simulink model "v06_arbitrary_coder"  (R2019b)
settings: Solver=FixedStepAuto  StartTime=0.0  StopTime=inf  FixedStep=1  MaxStep=1  RelTol=1e-3
libraries: simulink x3
settings Model: Creator=MARAT  LastModifiedBy=Marat
settings SFSimCC: CustomCodeUndefinedFunction=UseInterfaceOnly
settings ConfigComp: DVTestSuiteOptimization=Auto  DVDetectOutOfBounds=on

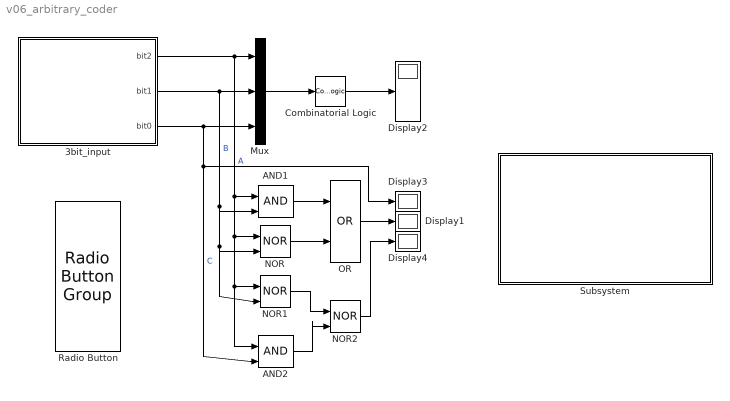
== system v06_arbitrary_coder ==
  3bit_input : Subsystem
      mask Display: image('images\3bit.jpg'); % Use "Edit Image" on toolstrip to change.
  AND1 : Logic  IconShape=distinctive  AllPortsSameDT=off  OutDataTypeStr=boolean
  AND2 : Logic  IconShape=distinctive  AllPortsSameDT=off  OutDataTypeStr=boolean
  Combinatorial Logic : CombinatorialLogic  TruthTable=[0 1 0 ; 1 1 0 ; 0 0 1 ; 1 0 1 ; 0 0 1 ; 1 0 0 ; 0 1 1 ; 1 1 0]
  Display{1..4} (4 alike) : Display
  Mux : Mux  Inputs=3
  NOR : Logic  Operator=NOR  IconShape=distinctive  AllPortsSameDT=off  OutDataTypeStr=boolean
  NOR1 : Logic  Operator=NOR  IconShape=distinctive  AllPortsSameDT=off  OutDataTypeStr=boolean
  NOR2 : Logic  Operator=NOR  IconShape=distinctive  AllPortsSameDT=off  OutDataTypeStr=boolean
  OR : Logic  Operator=OR  IconShape=distinctive  AllPortsSameDT=off  OutDataTypeStr=boolean
  Radio Button : RadioButtonGroup  SelectedLabel=0
      settings: Values={{'0', '1', '2', '3', '4', '5', '6', '7'}, [0 1 2 3 4 5 6 7]}
  Subsystem : Subsystem
      mask Display: image('D:\Work\DS_in_SL\pics\v06\table.png'); % Use "Edit Image" on toolstrip to change.
  wires:
  Mux/1 -> Combinatorial Logic/1
  Combinatorial Logic/1 -> Display2/1
  3bit_input/1(bit2) -> AND2/1, NOR1/1, NOR/1, AND1/1, Mux/1  "A"
  3bit_input/2(bit1) -> NOR1/2, NOR/2, AND1/2, Mux/2  "B"
  3bit_input/3(bit0) -> AND2/2, Display3/1, Mux/3  "C"
  AND1/1 -> OR/1
  OR/1 -> Display1/1
  NOR/1 -> OR/2
  NOR1/1 -> NOR2/1
  AND2/1 -> NOR2/2
  NOR2/1 -> Display4/1

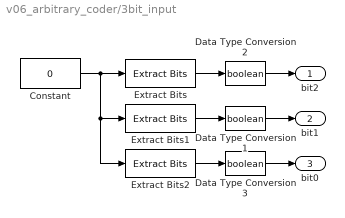
== system v06_arbitrary_coder/3bit_input ==
  Constant : Constant  Value=0  OutMin=0  OutMax=7  OutDataTypeStr=uint8
  Data Type Conversion1 : DataTypeConversion  OutDataTypeStr=boolean
  Data Type Conversion2 : DataTypeConversion  OutDataTypeStr=boolean
  Data Type Conversion3 : DataTypeConversion  OutDataTypeStr=boolean
  Extract Bits : simulink/Logic and Bit Operations/Extract Bits  bitsToExtract=Range of bits  numBits=8  bitIdxRange=2  outScalingMode=Treat bit field as an integer
      settings: SourceProductName=Simulink
  Extract Bits1 : simulink/Logic and Bit Operations/Extract Bits  bitsToExtract=Range of bits  numBits=8  bitIdxRange=1  outScalingMode=Treat bit field as an integer
      settings: SourceProductName=Simulink
  Extract Bits2 : simulink/Logic and Bit Operations/Extract Bits  bitsToExtract=Range of bits  numBits=8  bitIdxRange=0  outScalingMode=Treat bit field as an integer
      settings: SourceProductName=Simulink
  bit2 : Outport
  bit1 : Outport  Port=2
  bit0 : Outport  Port=3
  wires:
  Constant/1 -> Extract Bits2/1, Extract Bits1/1, Extract Bits/1
  Extract Bits/1 -> Data Type Conversion2/1
  Extract Bits1/1 -> Data Type Conversion1/1
  Extract Bits2/1 -> Data Type Conversion3/1
  Data Type Conversion2/1 -> bit2/1
  Data Type Conversion1/1 -> bit1/1
  Data Type Conversion3/1 -> bit0/1

== system v06_arbitrary_coder/Subsystem ==
